simulink model "Galvo_sys_Cdisc_Pcont_ccvc_FET_SUB_REF_v65"  (R2013a)
settings: Solver=ode23s  StartTime=0.0  StopTime=15e-3  FixedStep=FS  MaxStep=1e-4  RelTol=1e-3
PreLoadFcn:
  | vname=@(x) inputname(1);
  | paramCtrl=evalin('base','paramCtrl;');
  | I_LIM=str2num(paramCtrl.I_LIM);
  | Kbc=str2num(paramCtrl.Kbc);
  | FS=evalin('base','FS;');
InitFcn:
  | %%%%%%  set scope time range
  | T_STOP=str2num(get_param(gcs,'StopTime'));
  | if numel(T_STOP) > 1
  |    T_STOP=T_STOP(2);
  | else
  |    T_STOP=T_STOP(1);
  | end
  | T_STOP=num2str(T_STOP);
  | 
  | %%%%%%  set scope time range in system @init_callback_fct
  | T_STOP=num2str(str2num(get_param(gcs,'StopTime')));
  | 
  | childs = allchild(0);
  | sol=strfind(upper(get(allchild(0),'Tag')),'VIEWER_PARAMETERS');
  | 
  | if iscell(sol)
  |    ind=find(~cellfun(@isempty, strfind(upper(get(allchild(0),'Tag')),'VIEWER_PARAMETERS')));
  | else
  |    ind=sol;
  | end
  | %ind=find(~cellfun(@isempty, {strfind(upper(get(allchild(0),'Tag')),'VIEWER_PARAMETERS'),[]}))
  | if ~isempty(ind)
  |    for k=1:length(childs(ind))
  |       set_param(getfield(get(childs(ind(k)),'UserData'),'block'),'TimeRange',T_STOP);
  |       get_param(getfield(get(childs(ind(k)),'UserData'),'block'),'TimeRange');
  | %    set_param(getfield(get(childs(ind),'UserData'),'block'),'TimeRange',T_STOP);
  | %    get_param(getfield(get(childs(ind),'UserData'),'block'),'TimeRange');
  |    end
  | else
  |     warning(sprintf('VIEWER_PARAMETERS object not found\nOpen the config dialog by hand for the first sim start'))
  | end
StartFcn:
  | I_LIM=str2num(paramCtrl.I_LIM);
  | Kbc=str2num(paramCtrl.Kbc);
  | %FS=evalin('base','FS;');
values from neighbouring files (symbols this model uses):
  FB_EN = 1    [GalvoModel_v6_sys.m]    (also in Galvo_process_analyze.m = k-1; kompl_kreis_linmod_sensitiv.m)
  Lc = 170e-6    (= 0.00017)    [GalvoModel_v6_sys.m]    (also in Galvo_process_analyze.m)
  Rc = 1.5    [GalvoModel_v6_sys.m]    (also in Galvo_process_analyze.m; frequenzgang_nichtinvert_opamp_koblitz_eas.m = 1)
  Rsh = 0.003    [GalvoModel_v6_sys.m]    (also in Galvo_sys_proto_v13_OFFSETS_MODEL_PT1B_proc.m = 0.075; frequenzgang_nichtinvert_opamp_koblitz_eas.m = 0.015)
undefined symbols (not defined in the file or in its folder): ccG0, JR, KBM, KFR, KMT, KTB
libraries: simulink x5, dspsigops x1
Description:
  | Eigentlich sollte in diesem Modell als current comp. ein ref. block mit zwei Varianten "alte 12V endstufe" und "neue 30V endstufe" eingesetzt werden. Sobald ein subsystem als referenced model eingesetzt wird, kommen die warnungen wegen algebr. schleifen obwohl sich die Blockdiagramme nicht unterscheiden.
  | --> anstatt "referenced variants" kommt halt wieder ein "subsystem variants" block als
  | cc rein...
settings Model: BufferReuse=off  Creator=mainster  LastModifiedBy=mainster
settings SolverCC: AutoInsertRateTranBlk=on
settings DataIOCC: LimitDataPoints=off  SaveOutput=off  SaveTime=off
settings OptimizationCC: BlockReduction=off  InlineParams=on  OptimizeBlockIOStorage=off  BufferReuse=off  ExpressionFolding=off  LocalBlockOutputs=off
settings DebuggingCC: SolverPrmCheckMsg=none
settings ModelReferenceCC: ModelReferenceNumInstancesAllowed=Single  ModelReferenceMinAlgLoopOccurrences=on

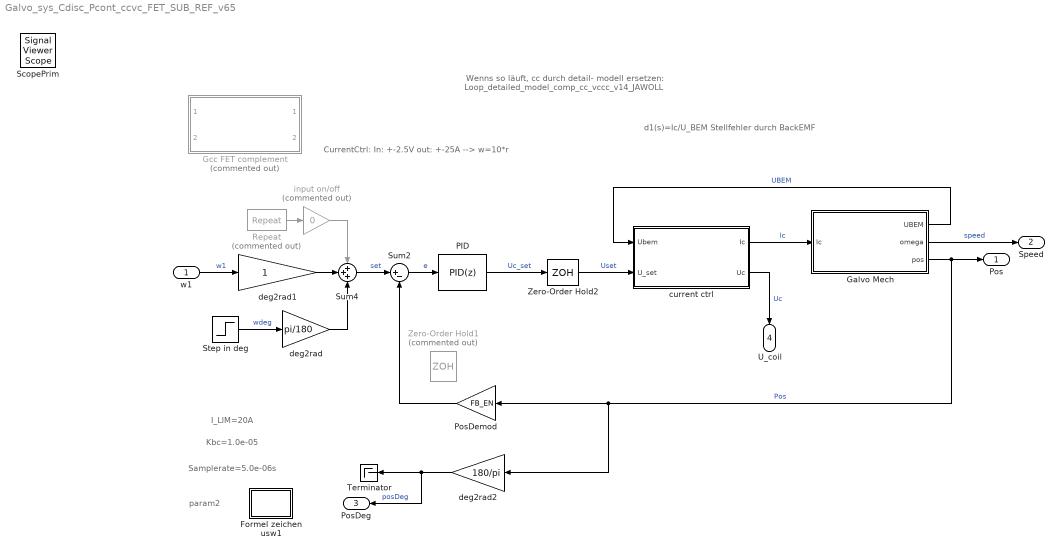
== system Galvo_sys_Cdisc_Pcont_ccvc_FET_SUB_REF_v65 ==
  note: I_LIM=20A
  note: Kbc=1.0e-05
  note: Samplerate=5.0e-06s
  note: d1(s)=Ic/U_BEM
      | Stellfehler durch BackEMF
  note: param2
  note: CurrentCtrl:
      | In:		+-2.5V
      | out: 	+-25A
      | --> w=10*r
  note: Wenns so läuft, cc durch detail- modell ersetzen:
      | Loop_detailed_model_comp_cc_vccc_v14_JAWOLL
  w1 : Inport
  Formel zeichen usw1 : Subsystem
  Galvo Mech : Subsystem
  Gcc FET complement : ModelReference  Commented=on  ModelNameDialog=CurrentComp_LR_estimated_old_pwr_b10.slx  SimulationMode=Normal  Variant=on  OverrideUsingVariant=estimated_cc  ModelReferenceVersion=1.450  CopyOfModelName=CurrentComp_LR_estimated_old_pwr_b10.slx  DefaultDataLogging=on
      mask Display:
      | str=sprintf('%s',get(gcbh,'ModelName'));
      | port_label('input', 1, 'U_{BEM}','texmode','on')
      | port_label('input', 2, 'I/U_{Set}','texmode','on')
      | port_label('output', 1, 'I_{Coil}','texmode','on')
      | port_label('output', 2, 'U_{Coil}','texmode','on')
      | %text(.05,.98,['{\fontsize{12}\it\bf' strrep(str,'_',' ') '}'],'horizontalAlignment','left','verticalAlignment','top','texmode','on')
      | text(.5,0.95,['{\fontsize{12}\it\bfG_{cc}(s)}'],'horizontalAlignment','center','verticalAlignment','top','texmode','on')
      | text(.5,0.65,['{\fontsize{14}\it\bfFET v1}'],'horizontalAlignment','center','verticalAlignment','top','texmode','on')
      | %text(.15,.05,['{\fontsize{10}\itmechanics}'],'horizontalAlignment','left','verticalAlignment','bottom','texmode','on')
  PID : simulink/Continuous/PID Controller  OverrideUsingVariant=Ccc_no_vc  Controller=PID  TimeDomain=Discrete-time  SampleTime=FS  IntegratorMethod=Forward Euler  FilterMethod=Forward Euler  Form=Parallel  P=0.388587122152474  I=1.78014614654243  D=0.000908843135465162  N=1093.06989088429  InitialConditionSource=internal  InitialConditionForIntegrator=0  InitialConditionForFilter=0  ExternalReset=none  IgnoreLimit=on  LimitOutput=on  UpperSaturationLimit=30  LowerSaturationLimit=-30  LinearizeAsGain=off  AntiWindupMode=clamping  Kb=0.1  TrackingMode=off  Kt=0  PParamMin=[]  PParamMax=[]  IParamMin=[]  IParamMax=[]  DParamMin=[]  DParamMax=[]  NParamMin=[]  NParamMax=[]  KbParamMin=[]  KbParamMax=[]  KtParamMin=[]  KtParamMax=[]  POutMin=[]  POutMax=[]  IOutMin=[]  IOutMax=[]  DOutMin=[]  DOutMax=[]  NOutMin=[]  NOutMax=[]  KbOutMin=[]  KbOutMax=[]  KtOutMin=[]  KtOutMax=[]  IntegratorOutMin=[]  IntegratorOutMax=[]  FilterOutMin=[]  FilterOutMax=[]  SumOutMin=[]  SumOutMax=[]  SumI1OutMin=[]  SumI1OutMax=[]  SumI2OutMin=[]  SumI2OutMax=[]  SumI3OutMin=[]  SumI3OutMax=[]  SumDOutMin=[]  SumDOutMax=[]  SaturationOutMin=[]  SaturationOutMax=[]  IntegratorContinuousStateAttributes=''  IntegratorStateMustResolveToSignalObject=off  IntegratorRTWStateStorageClass=Auto  FilterContinuousStateAttributes=''  FilterStateMustResolveToSignalObject=off  FilterRTWStateStorageClass=Auto
      settings: AttributesFormatString=UpLim:%<UpperSaturationLimit>\nLoLim:%<LowerSaturationLimit>
  PosDemod : Gain  Gain=FB_EN
  Repeat : dspsigops/Repeat  Commented=on  N=length(str2num(get_param([gcs '/Sequence Stair'], 'OutValues')))  InputProcessing=Columns as channels (frame based)  RateOptions=Allow multirate processing  ic=0  mode=Unused parameter value
  Step in deg : Step  Time=1e-3  After=5  SampleTime=FS  ZeroCross=off
      settings: AttributesFormatString=Ampl.: %<After>\ntime:%<Time>
  Sum2 : Sum  Inputs=|+-
  Sum4 : Sum  Inputs=+++  SampleTime=FS
  Terminator : Terminator
  Zero-Order Hold1 : ZeroOrderHold  Commented=on  SampleTime=FS
  Zero-Order Hold2 : ZeroOrderHold  SampleTime=FS
  current ctrl : Subsystem  Variant=on  OverrideUsingVariant=Ccc_blocks_est
  deg2rad : Gain  Gain=pi/180  SampleTime=FS
  deg2rad1 : Gain  SampleTime=FS
  deg2rad2 : Gain  Gain=180/pi
  input on/off : Gain  Commented=on  Gain=0  SampleTime=FS
  Pos : Outport
  Speed : Outport  Port=2
  PosDeg : Outport  Port=3
  U_coil : Outport  Port=4
  ScopePrim : SignalViewerScope  IOType=viewer  NumInputPorts=5  LegendLocations=|  RefreshTime=0.033391
      | 0.77537     0.92196     0.16697    0.037382
      | 0.77537     0.74948     0.16697    0.020986
      | 0.81965     0.55955     0.12269    0.020986
      | 0.78644     0.37067     0.12269    0.020986
      |       0           0           0           0
      settings: ShowLegends=on  TimeRange=0.015  YMin=0~-0.05~-1.5~-0.1~-0.5  YMax=6~0.15~1~0.3~2
  wires:
  w1/1 -> deg2rad1/1  "w1"
  Repeat/1 -> input on/off/1
  Sum2/1 -> PID/1  "e"
  Sum4/1 -> Sum2/1  "set"
  Step in deg/1 -> deg2rad/1  "wdeg"
  input on/off/1 -> Sum4/1
  deg2rad/1 -> Sum4/3
  deg2rad2/1 -> PosDeg/1, Terminator/1  "posDeg"
  deg2rad1/1 -> Sum4/2
  PosDemod/1 -> Sum2/2
  PID/1 -> Zero-Order Hold2/1  "Uc_set"
  Zero-Order Hold2/1 -> current ctrl/2(U_set)  "Uset"
  current ctrl/2(Uc) -> U_coil/1  "Uc"
  Galvo Mech/3(pos) -> deg2rad2/1, PosDemod/1, Pos/1  "Pos"
  current ctrl/1(Ic) -> Galvo Mech/1(Ic)  "Ic"
  Galvo Mech/2(omega) -> Speed/1  "speed"
  Galvo Mech/1(UBEM) -> current ctrl/1(Ubem)  "UBEM"

== system Galvo_sys_Cdisc_Pcont_ccvc_FET_SUB_REF_v65/Formel zeichen usw1 ==
  note: Te: 		electrical torque, gen. by coils		[Nm]
      |  Ic: 			coil current							[A]
      |  Tfr:		rotor dynamic friction torque 		[Nm]
      |  Trb:		torsion bar torque					[Nm]
      |  Tw:		angular momentum				[Nm*s]
      |  w:			angular velocity 					[rad/s]
      |  yrad:		angular position 					[rad]
      |  ydeg:		angular position 					[°]
      |  Ucci:		current controller input				[V]
      |  Ucco:		current controller output			[V]
      |  Ush:		shunt voltage						[V]
  note: L_{c  }	coil inductance 							[H]
      |  R_{c  }	coil resistance							[\Omega]
      |  R_{SH }	current shunt resistance				[\Omega]
      |  J_{R  }	rotor inertia 							[kg*m²]
      |  K_{TB }	torsion bar torque const. 			[Nm/rad]
      |  K_{BM }	back EMF const.							[V*s/rad]
      |  K_{FR }	rotor dyn. friction torque const.	[Nm*s/rad]
      |  K_{MT }	el. magnetic torque const.			[Nm/A]
  note: balance of force: 	Te=Ttb+Tfr
      | 					Te - (Ttb+Tfr)=0  ->  no movement
      |
      |  integrate( 1 Nm )dt = 1 Nm*s
      |  (Nm*s)(kg*m²)⁻¹ = (N*s/kg)*m⁻¹ = m/(s*m) = rad

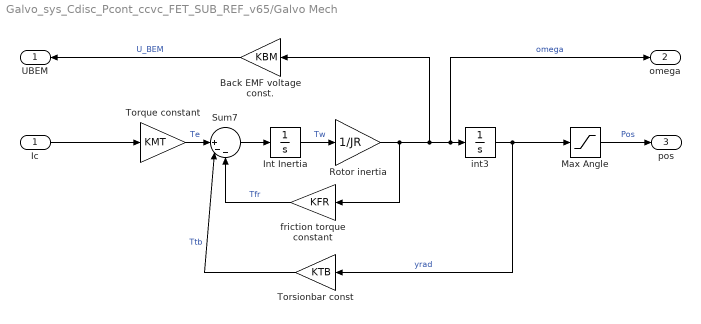
== system Galvo_sys_Cdisc_Pcont_ccvc_FET_SUB_REF_v65/Galvo Mech ==
  Ic : Inport
  Back EMF voltage const. : Gain  Gain=KBM
  Int Inertia : Integrator
  Max Angle : Saturate  UpperLimit=20*pi/180  LowerLimit=-20*pi/180
      settings: AttributesFormatString=Max=%<UpperLimit>\nMin=%<LowerLimit>
  Rotor inertia : Gain  Gain=1/JR
  Sum7 : Sum  Inputs=||+--
  Torque constant : Gain  Gain=KMT
  Torsionbar const : Gain  Gain=KTB
  friction torque constant : Gain  Gain=KFR
  int3 : Integrator
  UBEM : Outport
  omega : Outport  Port=2
  pos : Outport  Port=3
  wires:
  Int Inertia/1 -> Rotor inertia/1  "Tw"
  Max Angle/1 -> pos/1  "Pos"
  Torsionbar const/1 -> Sum7/2  "Ttb"
  Sum7/1 -> Int Inertia/1
  Back EMF voltage const./1 -> UBEM/1  "U_BEM"
  int3/1 -> Max Angle/1, Torsionbar const/1  "yrad"
  Rotor inertia/1 -> omega/1, int3/1, Back EMF voltage const./1, friction torque constant/1  "omega"
  Torque constant/1 -> Sum7/1  "Te"
  friction torque constant/1 -> Sum7/3  "Tfr"
  Ic/1 -> Torque constant/1

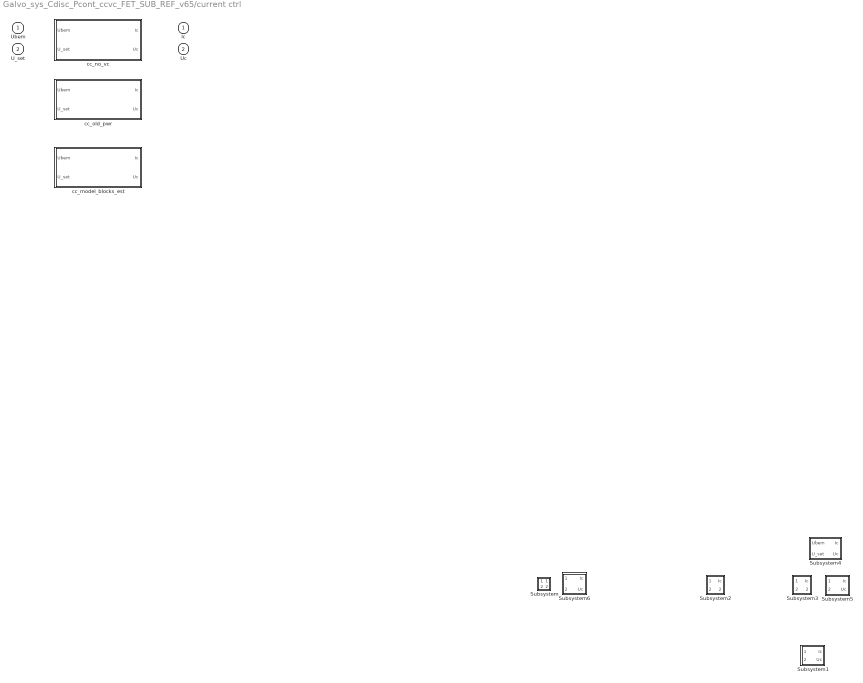
== system Galvo_sys_Cdisc_Pcont_ccvc_FET_SUB_REF_v65/current ctrl ==
  Ubem : Inport
  U_set : Inport  Port=2
  Subsystem : Subsystem  VariantControl=Variant
  Subsystem1 : Subsystem  VariantControl=Variant2
  Subsystem2 : Subsystem  VariantControl=Variant3
  Subsystem3 : Subsystem  VariantControl=Variant4
  Subsystem4 : Subsystem  VariantControl=Variant5
  Subsystem5 : Subsystem  VariantControl=Variant6
  Subsystem6 : Subsystem  VariantControl=Variant7
  cc_model_blocks_est : Subsystem  VariantControl=Ccc_blocks_est
  cc_no_vc : Subsystem  VariantControl=Ccc_no_vc
  cc_old_pwr : Subsystem  VariantControl=Ccc_old_pwr
  Ic : Outport
  Uc : Outport  Port=2

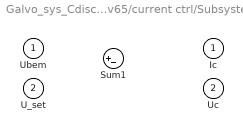
== system Galvo_sys_Cdisc_Pcont_ccvc_FET_SUB_REF_v65/current ctrl/Subsystem ==
  Ubem : Inport
  U_set : Inport  Port=2
  Sum1 : Sum  Inputs=|+-
  Ic : Outport
  Uc : Outport  Port=2

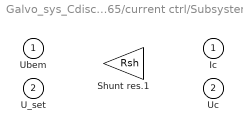
== system Galvo_sys_Cdisc_Pcont_ccvc_FET_SUB_REF_v65/current ctrl/Subsystem1 ==
  Ubem : Inport
  U_set : Inport  Port=2
  Shunt res.1 : Gain  Gain=Rsh
  Ic : Outport
  Uc : Outport  Port=2

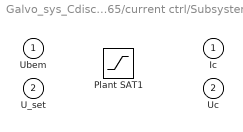
== system Galvo_sys_Cdisc_Pcont_ccvc_FET_SUB_REF_v65/current ctrl/Subsystem2 ==
  Ubem : Inport
  U_set : Inport  Port=2
  Plant SAT1 : Saturate  UpperLimit=15  LowerLimit=-15
      settings: AttributesFormatString=U_lim=+-%<UpperLimit>V
  Ic : Outport
  Uc : Outport  Port=2

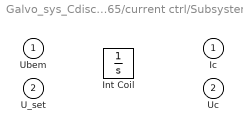
== system Galvo_sys_Cdisc_Pcont_ccvc_FET_SUB_REF_v65/current ctrl/Subsystem3 ==
  Ubem : Inport
  U_set : Inport  Port=2
  Int Coil : Integrator
  Ic : Outport
  Uc : Outport  Port=2

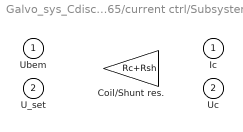
== system Galvo_sys_Cdisc_Pcont_ccvc_FET_SUB_REF_v65/current ctrl/Subsystem4 ==
  Ubem : Inport
  U_set : Inport  Port=2
  Coil/Shunt res. : Gain  Gain=Rc+Rsh
  Ic : Outport
  Uc : Outport  Port=2

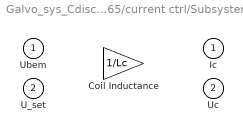
== system Galvo_sys_Cdisc_Pcont_ccvc_FET_SUB_REF_v65/current ctrl/Subsystem5 ==
  Ubem : Inport
  U_set : Inport  Port=2
  Coil Inductance : Gain  Gain=1/Lc
  Ic : Outport
  Uc : Outport  Port=2

== system Galvo_sys_Cdisc_Pcont_ccvc_FET_SUB_REF_v65/current ctrl/Subsystem6 ==
  Ubem : Inport
  U_set : Inport  Port=2
  Cc(s) : simulink/Continuous/PID Controller  Controller=P  TimeDomain=Continuous-time  SampleTime=-1  IntegratorMethod=Forward Euler  FilterMethod=Forward Euler  Form=Ideal  P=3.52446212597481  I=14078.2261040339  D=0  N=100  InitialConditionSource=internal  InitialConditionForIntegrator=0  InitialConditionForFilter=0  ExternalReset=none  LimitOutput=off  UpperSaturationLimit=inf  LowerSaturationLimit=-inf  LinearizeAsGain=on  AntiWindupMode=none  Kb=1  TrackingMode=off  Kt=1  PParamMin=[]  PParamMax=[]  IParamMin=[]  IParamMax=[]  DParamMin=[]  DParamMax=[]  NParamMin=[]  NParamMax=[]  KbParamMin=[]  KbParamMax=[]  KtParamMin=[]  KtParamMax=[]  POutMin=[]  POutMax=[]  IOutMin=[]  IOutMax=[]  DOutMin=[]  DOutMax=[]  NOutMin=[]  NOutMax=[]  KbOutMin=[]  KbOutMax=[]  KtOutMin=[]  KtOutMax=[]  IntegratorOutMin=[]  IntegratorOutMax=[]  FilterOutMin=[]  FilterOutMax=[]  SumOutMin=[]  SumOutMax=[]  SumI1OutMin=[]  SumI1OutMax=[]  SumI2OutMin=[]  SumI2OutMax=[]  SumI3OutMin=[]  SumI3OutMax=[]  SumDOutMin=[]  SumDOutMax=[]  SaturationOutMin=[]  SaturationOutMax=[]  IntegratorContinuousStateAttributes=''  IntegratorStateMustResolveToSignalObject=off  IntegratorRTWStateStorageClass=Auto  FilterContinuousStateAttributes=''  FilterStateMustResolveToSignalObject=off  FilterRTWStateStorageClass=Auto
  Ic : Outport
  Uc : Outport  Port=2

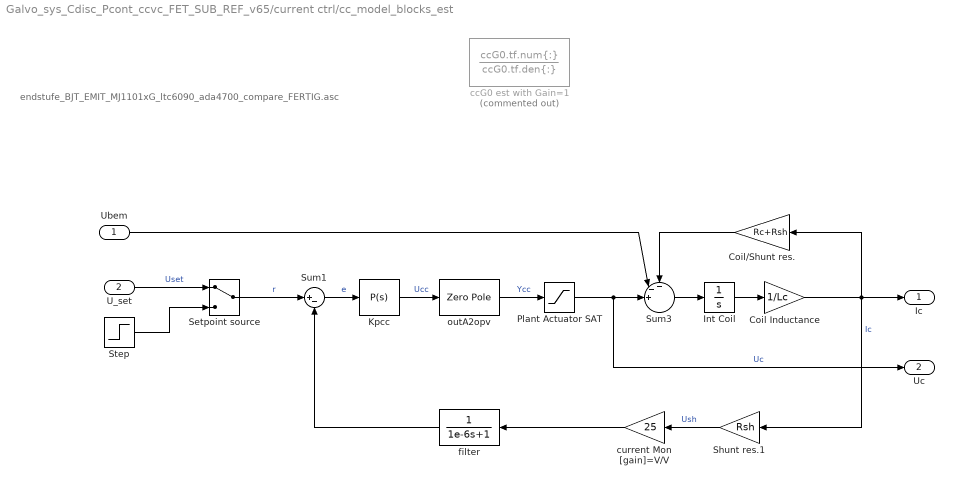
== system Galvo_sys_Cdisc_Pcont_ccvc_FET_SUB_REF_v65/current ctrl/cc_model_blocks_est ==
  note: endstufe_BJT_EMIT_MJ1101xG_ltc6090_ada4700_compare_FERTIG.asc
  Ubem : Inport
  U_set : Inport  Port=2
  Coil Inductance : Gain  Gain=1/Lc
  Coil/Shunt res. : Gain  Gain=Rc+Rsh
  Int Coil : Integrator
  Kpcc : simulink/Continuous/PID Controller  Controller=P  TimeDomain=Continuous-time  SampleTime=-1  IntegratorMethod=Forward Euler  FilterMethod=Forward Euler  Form=Ideal  P=16.17  I=14078.2261040339  D=0  N=100  InitialConditionSource=internal  InitialConditionForIntegrator=0  InitialConditionForFilter=0  ExternalReset=none  LimitOutput=off  UpperSaturationLimit=inf  LowerSaturationLimit=-inf  LinearizeAsGain=on  AntiWindupMode=none  Kb=1  TrackingMode=off  Kt=1  PParamMin=[]  PParamMax=[]  IParamMin=[]  IParamMax=[]  DParamMin=[]  DParamMax=[]  NParamMin=[]  NParamMax=[]  KbParamMin=[]  KbParamMax=[]  KtParamMin=[]  KtParamMax=[]  POutMin=[]  POutMax=[]  IOutMin=[]  IOutMax=[]  DOutMin=[]  DOutMax=[]  NOutMin=[]  NOutMax=[]  KbOutMin=[]  KbOutMax=[]  KtOutMin=[]  KtOutMax=[]  IntegratorOutMin=[]  IntegratorOutMax=[]  FilterOutMin=[]  FilterOutMax=[]  SumOutMin=[]  SumOutMax=[]  SumI1OutMin=[]  SumI1OutMax=[]  SumI2OutMin=[]  SumI2OutMax=[]  SumI3OutMin=[]  SumI3OutMax=[]  SumDOutMin=[]  SumDOutMax=[]  SaturationOutMin=[]  SaturationOutMax=[]  IntegratorContinuousStateAttributes=''  IntegratorStateMustResolveToSignalObject=off  IntegratorRTWStateStorageClass=Auto  FilterContinuousStateAttributes=''  FilterStateMustResolveToSignalObject=off  FilterRTWStateStorageClass=Auto
      settings: AttributesFormatString=Kp=%<P>
  Plant Actuator SAT : Saturate  UpperLimit=150  LowerLimit=-150
      settings: AttributesFormatString=U_lim=+-%<UpperLimit>V
  Setpoint source : ManualSwitch
  Shunt res.1 : Gain  Gain=Rsh
  Step : Step  SampleTime=0
  Sum1 : Sum  Inputs=|+-
  Sum3 : Sum  Inputs=--+||
  ccG0 est with Gain=1 : TransferFcn  Commented=on  Numerator=ccG0.tf.num{:}  Denominator=ccG0.tf.den{:}
      settings: AttributesFormatString=%<numerator>\n%<denominator>
  current Mon [gain]=V/V : Gain  Gain=25
  filter : TransferFcn  Denominator=[1e-6 1]
  outA2opv : ZeroPole  Zeros=3.4653e+08  Poles=-2.6678e+08  Gain=-0.7684
  Ic : Outport
  Uc : Outport  Port=2
  wires:
  outA2opv/1 -> Plant Actuator SAT/1  "Ycc"
  Sum1/1 -> Kpcc/1  "e"
  Coil Inductance/1 -> Ic/1, Shunt res.1/1, Coil/Shunt res./1  "Ic"
  Plant Actuator SAT/1 -> Uc/1, Sum3/3  "Uc"
  Coil/Shunt res./1 -> Sum3/1
  Sum3/1 -> Int Coil/1
  Int Coil/1 -> Coil Inductance/1
  Shunt res.1/1 -> current Mon [gain]=V/V/1  "Ush"
  current Mon [gain]=V/V/1 -> filter/1
  Ubem/1 -> Sum3/2
  U_set/1 -> Setpoint source/1  "Uset"
  Step/1 -> Setpoint source/2
  Setpoint source/1 -> Sum1/1  "r"
  Kpcc/1 -> outA2opv/1  "Ucc"
  filter/1 -> Sum1/2

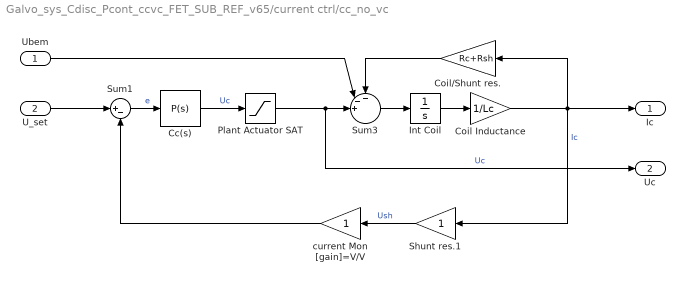
== system Galvo_sys_Cdisc_Pcont_ccvc_FET_SUB_REF_v65/current ctrl/cc_no_vc ==
  Ubem : Inport
  U_set : Inport  Port=2
  Cc(s) : simulink/Continuous/PID Controller  Controller=P  TimeDomain=Continuous-time  SampleTime=-1  IntegratorMethod=Forward Euler  FilterMethod=Forward Euler  Form=Ideal  P=6.3432542926282  I=14078.2261040339  D=0  N=100  InitialConditionSource=internal  InitialConditionForIntegrator=0  InitialConditionForFilter=0  ExternalReset=none  LimitOutput=off  UpperSaturationLimit=inf  LowerSaturationLimit=-inf  LinearizeAsGain=on  AntiWindupMode=none  Kb=1  TrackingMode=off  Kt=1  PParamMin=[]  PParamMax=[]  IParamMin=[]  IParamMax=[]  DParamMin=[]  DParamMax=[]  NParamMin=[]  NParamMax=[]  KbParamMin=[]  KbParamMax=[]  KtParamMin=[]  KtParamMax=[]  POutMin=[]  POutMax=[]  IOutMin=[]  IOutMax=[]  DOutMin=[]  DOutMax=[]  NOutMin=[]  NOutMax=[]  KbOutMin=[]  KbOutMax=[]  KtOutMin=[]  KtOutMax=[]  IntegratorOutMin=[]  IntegratorOutMax=[]  FilterOutMin=[]  FilterOutMax=[]  SumOutMin=[]  SumOutMax=[]  SumI1OutMin=[]  SumI1OutMax=[]  SumI2OutMin=[]  SumI2OutMax=[]  SumI3OutMin=[]  SumI3OutMax=[]  SumDOutMin=[]  SumDOutMax=[]  SaturationOutMin=[]  SaturationOutMax=[]  IntegratorContinuousStateAttributes=''  IntegratorStateMustResolveToSignalObject=off  IntegratorRTWStateStorageClass=Auto  FilterContinuousStateAttributes=''  FilterStateMustResolveToSignalObject=off  FilterRTWStateStorageClass=Auto
  Coil Inductance : Gain  Gain=1/Lc
  Coil/Shunt res. : Gain  Gain=Rc+Rsh
  Int Coil : Integrator
  Plant Actuator SAT : Saturate  UpperLimit=30  LowerLimit=-30
      settings: AttributesFormatString=U_lim=+-%<UpperLimit>A
  Shunt res.1 : Gain
  Sum1 : Sum  Inputs=|+-
  Sum3 : Sum  Inputs=--+||
  current Mon [gain]=V/V : Gain
  Ic : Outport
  Uc : Outport  Port=2
  wires:
  Sum3/1 -> Int Coil/1
  Cc(s)/1 -> Plant Actuator SAT/1  "Uc"
  Coil/Shunt res./1 -> Sum3/1
  Ubem/1 -> Sum3/2
  Int Coil/1 -> Coil Inductance/1
  Coil Inductance/1 -> Coil/Shunt res./1, Shunt res.1/1, Ic/1  "Ic"
  Shunt res.1/1 -> current Mon [gain]=V/V/1  "Ush"
  Plant Actuator SAT/1 -> Sum3/3, Uc/1  "Uc"
  U_set/1 -> Sum1/1
  current Mon [gain]=V/V/1 -> Sum1/2
  Sum1/1 -> Cc(s)/1  "e"

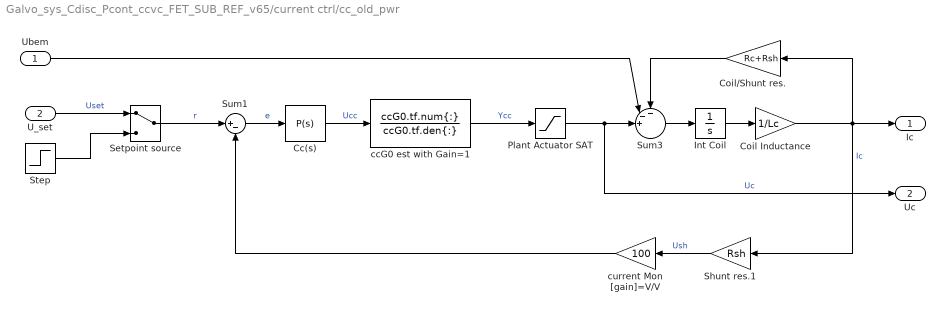
== system Galvo_sys_Cdisc_Pcont_ccvc_FET_SUB_REF_v65/current ctrl/cc_old_pwr ==
  Ubem : Inport
  U_set : Inport  Port=2
  Cc(s) : simulink/Continuous/PID Controller  Controller=P  TimeDomain=Continuous-time  SampleTime=-1  IntegratorMethod=Forward Euler  FilterMethod=Forward Euler  Form=Ideal  P=3.52446212597481  I=14078.2261040339  D=0  N=100  InitialConditionSource=internal  InitialConditionForIntegrator=0  InitialConditionForFilter=0  ExternalReset=none  LimitOutput=off  UpperSaturationLimit=inf  LowerSaturationLimit=-inf  LinearizeAsGain=on  AntiWindupMode=none  Kb=1  TrackingMode=off  Kt=1  PParamMin=[]  PParamMax=[]  IParamMin=[]  IParamMax=[]  DParamMin=[]  DParamMax=[]  NParamMin=[]  NParamMax=[]  KbParamMin=[]  KbParamMax=[]  KtParamMin=[]  KtParamMax=[]  POutMin=[]  POutMax=[]  IOutMin=[]  IOutMax=[]  DOutMin=[]  DOutMax=[]  NOutMin=[]  NOutMax=[]  KbOutMin=[]  KbOutMax=[]  KtOutMin=[]  KtOutMax=[]  IntegratorOutMin=[]  IntegratorOutMax=[]  FilterOutMin=[]  FilterOutMax=[]  SumOutMin=[]  SumOutMax=[]  SumI1OutMin=[]  SumI1OutMax=[]  SumI2OutMin=[]  SumI2OutMax=[]  SumI3OutMin=[]  SumI3OutMax=[]  SumDOutMin=[]  SumDOutMax=[]  SaturationOutMin=[]  SaturationOutMax=[]  IntegratorContinuousStateAttributes=''  IntegratorStateMustResolveToSignalObject=off  IntegratorRTWStateStorageClass=Auto  FilterContinuousStateAttributes=''  FilterStateMustResolveToSignalObject=off  FilterRTWStateStorageClass=Auto
  Coil Inductance : Gain  Gain=1/Lc
  Coil/Shunt res. : Gain  Gain=Rc+Rsh
  Int Coil : Integrator
  Plant Actuator SAT : Saturate  UpperLimit=15  LowerLimit=-15
      settings: AttributesFormatString=U_lim=+-%<UpperLimit>V
  Setpoint source : ManualSwitch
  Shunt res.1 : Gain  Gain=Rsh
  Step : Step  SampleTime=0
  Sum1 : Sum  Inputs=|+-
  Sum3 : Sum  Inputs=--+||
  ccG0 est with Gain=1 : TransferFcn  Numerator=ccG0.tf.num{:}  Denominator=ccG0.tf.den{:}
      settings: AttributesFormatString=%<numerator>\n%<denominator>
  current Mon [gain]=V/V : Gain  Gain=100
  Ic : Outport
  Uc : Outport  Port=2
  wires:
  ccG0 est with Gain=1/1 -> Plant Actuator SAT/1  "Ycc"
  Sum1/1 -> Cc(s)/1  "e"
  Coil Inductance/1 -> Ic/1, Shunt res.1/1, Coil/Shunt res./1  "Ic"
  Plant Actuator SAT/1 -> Uc/1, Sum3/3  "Uc"
  Coil/Shunt res./1 -> Sum3/1
  Sum3/1 -> Int Coil/1
  Int Coil/1 -> Coil Inductance/1
  Cc(s)/1 -> ccG0 est with Gain=1/1  "Ucc"
  Shunt res.1/1 -> current Mon [gain]=V/V/1  "Ush"
  current Mon [gain]=V/V/1 -> Sum1/2
  Ubem/1 -> Sum3/2
  U_set/1 -> Setpoint source/1  "Uset"
  Step/1 -> Setpoint source/2
  Setpoint source/1 -> Sum1/1  "r"
